simulink model "ej4"  (R2020b)
settings: Solver=ode4  StartTime=0.0  StopTime=30.0  FixedStep=0.05  RelTol=1e-3
settings Model: Creator=Kike  LastModifiedBy=zunt7

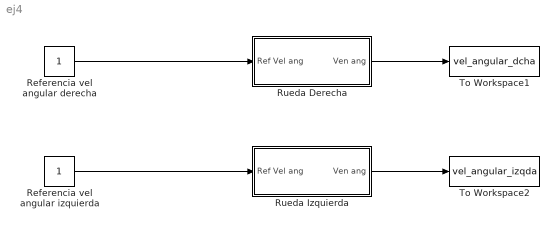
== system ej4 ==
  Referencia vel angular derecha : Constant
  Referencia vel angular izquierda : Constant
  Rueda Derecha : Subsystem  mask{k=0.2, tau=0.09, kp=3}
      mask prompts: k "Valor ganancia motor:"; tau "Valor cte tiempo motor:"; kp "Valor ganancia regulador P:"
  Rueda Izquierda : Subsystem  mask{tau=0.09, kp=3, k=0.2}
      mask prompts: tau "Valor cte tiempo motor:"; kp "Valor ganancia regulador P:"; k "Valor ganancia motor:"
  To Workspace1 : ToWorkspace  VariableName=vel_angular_dcha  SaveFormat=Timeseries  SampleTime=-1
  To Workspace2 : ToWorkspace  VariableName=vel_angular_izqda  SaveFormat=Timeseries  SampleTime=-1
  wires:
  Referencia vel angular derecha/1 -> Rueda Derecha/1(Ref Vel ang)
  Rueda Derecha/1(Ven ang) -> To Workspace1/1
  Rueda Izquierda/1(Ven ang) -> To Workspace2/1
  Referencia vel angular izquierda/1 -> Rueda Izquierda/1(Ref Vel ang)

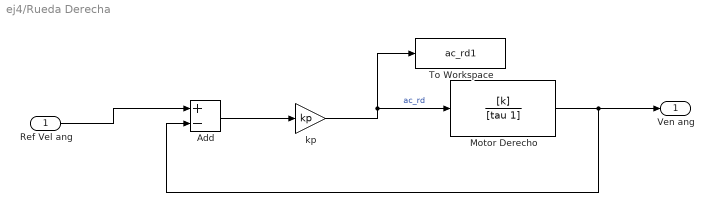
== system ej4/Rueda Derecha ==
  Ref Vel ang : Inport
  Add : Sum  Inputs=+-
  Motor Derecho : TransferFcn  Numerator=[k]  Denominator=[tau 1]
  To Workspace : ToWorkspace  VariableName=ac_rd1  SaveFormat=Timeseries  SampleTime=-1
  kp : Gain  Gain=kp
  Ven ang : Outport
  wires:
  Ref Vel ang/1 -> Add/1
  kp/1 -> To Workspace/1, Motor Derecho/1  "ac_rd"
  Add/1 -> kp/1
  Motor Derecho/1 -> Add/2, Ven ang/1

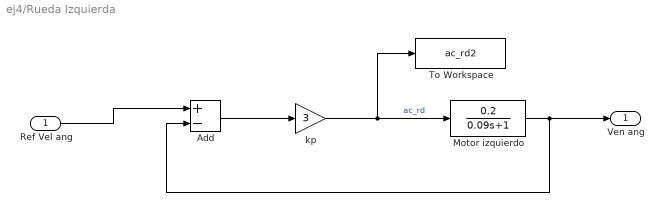
== system ej4/Rueda Izquierda ==
  Ref Vel ang : Inport
  Add : Sum  Inputs=+-
  Motor izquierdo : TransferFcn  Numerator=[0.2]  Denominator=[0.09 1]
  To Workspace : ToWorkspace  VariableName=ac_rd2  SaveFormat=Timeseries  SampleTime=-1
  kp : Gain  Gain=3
  Ven ang : Outport
  wires:
  Ref Vel ang/1 -> Add/1
  kp/1 -> To Workspace/1, Motor izquierdo/1  "ac_rd"
  Add/1 -> kp/1
  Motor izquierdo/1 -> Ven ang/1, Add/2
